simulink model "untitled"  (R2021b)
settings: Solver=VariableStepAuto  StartTime=0.0  StopTime=10.0  RelTol=1e-3
settings Model: Creator=Mazen  LastModifiedBy=Mazen
settings DebuggingCC: UnconnectedInputMsg=none  UnconnectedOutputMsg=none  UnconnectedLineMsg=none
settings ModelReferenceCC: EnableRefExpFcnMdlSchedulingChecks=off
settings RTWCC: DLArmComputeVersion=20.02.1

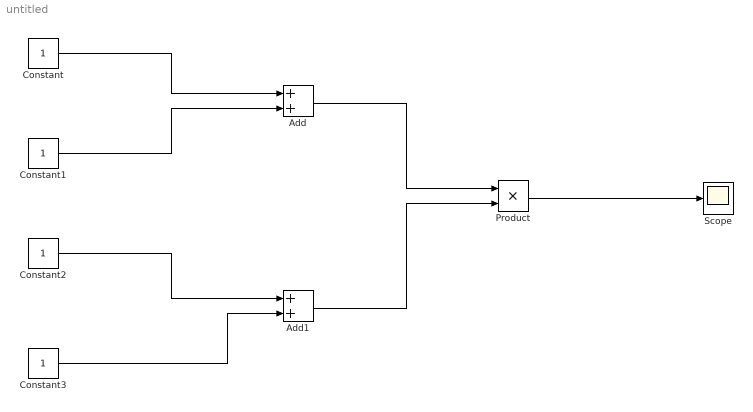
== system untitled ==
  Add : Sum
  Add1 : Sum
  Constant{,1..3} (4 alike) : Constant
  Product : Product
  Scope : Scope
  wires:
  Constant/1 -> Add/1
  Constant1/1 -> Add/2
  Constant2/1 -> Add1/1
  Constant3/1 -> Add1/2
  Add/1 -> Product/1
  Add1/1 -> Product/2
  Product/1 -> Scope/1
